simulink model "system66"  (R2021a)
settings: Solver=VariableStepAuto  StartTime=0.0  StopTime=StopTime  RelTol=1e-3
values from neighbouring files (symbols this model uses):
  A = [-0.003 0.039 0 -0.322; -0.065 -0.319 7.74 0; 0.020 -0.101 -0.429 0; 0 0 1 0]    [test_2_2_system.m]    (also in test_6_outputs_8_inputs_identification.m = [-0.01 2.2 3.3 4.4 5.5 6.6)
  Ad = sys_dt.A    [test_2_2_system.m]    (also in test_6_outputs_8_inputs_identification.m)
  B = [0.010 1; -0.18 -0.04; -1.16 0.598; 0 0]    [test_2_2_system.m]    (also in test_6_outputs_8_inputs_identification.m = rand(6,6))
  Bd = sys_dt.B    [test_2_2_system.m]    (also in test_6_outputs_8_inputs_identification.m)
  C = [1 0 0 0; 0 -1 0 7.74]    [test_2_2_system.m]    (also in test_6_outputs_8_inputs_identification.m = rand(6,6))
  Cd = sys_dt.C    [test_2_2_system.m]    (also in test_6_outputs_8_inputs_identification.m)
  D = zeros(2,2)    [test_2_2_system.m]    (also in test_6_outputs_8_inputs_identification.m = zeros(6,6))
  Dd = sys_dt.D    [test_2_2_system.m]    (also in test_6_outputs_8_inputs_identification.m)
  Ts = 1/fs    [NAPAS_closed_loop.m]    (also in NAPAS_closed_loop_T_and_S.m; test_2_2_system.m; test_6_outputs_8_inputs_identification.m; test_multisine.m)
settings Model: Creator=42447  LastModifiedBy=42447

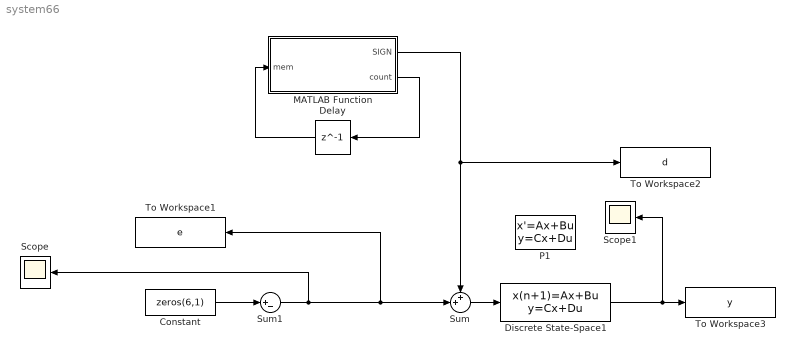
== system system66 ==
  Constant : Constant  Value=zeros(6,1)
  Delay : Delay  DelayLength=1  InitialCondition=1  SampleTime=Ts
  Discrete State-Space1 : DiscreteStateSpace  A=Ad  B=Bd  C=Cd  D=Dd  SampleTime=-1
  MATLAB Function : MATLAB Function  TreatAsAtomicUnit=on
  P1 : StateSpace  A=A  B=B  C=C  D=D  InitialCondition=0
  Scope : Scope
  Scope1 : Scope
  Sum : Sum  Inputs=++|
  Sum1 : Sum  Inputs=|+-
  To Workspace1 : ToWorkspace  VariableName=e  SaveFormat=Structure With Time  SampleTime=-1
  To Workspace2 : ToWorkspace  VariableName=d  SaveFormat=Structure With Time  SampleTime=-1
  To Workspace3 : ToWorkspace  VariableName=y  SaveFormat=Structure With Time  SampleTime=-1
  wires:
  Discrete State-Space1/1 -> Scope1/1, To Workspace3/1
  Sum/1 -> Discrete State-Space1/1
  MATLAB Function/1(SIGN) -> Sum/1, To Workspace2/1
  Constant/1 -> Sum1/1
  Sum1/1 -> Sum/2, To Workspace1/1, Scope/1
  MATLAB Function/2(count) -> Delay/1
  Delay/1 -> MATLAB Function/1(mem)

== matlab function system66/MATLAB Function ==
  data: SIGN output; mem input; count output; EXCSIG parameter
function [SIGN,count] = fcn(mem, EXCSIG)

SIGN    =   EXCSIG(:,mem);
count   =   mem + 1;
